simulink model "rbc_ut"  (Simulink 8.1)
settings: Solver=FixedStepDiscrete  StartTime=0.0  StopTime=Inf  FixedStep=0.005  RelTol=1e-3
PostLoadFcn:
  | , if any(exist('dsrtsu_mdlpostloadfcn', 'file') == [2, 3, 6]), try dsrtsu_mdlpostloadfcn('Execute', bdroot); catch fprintf('Error in PostLoadFcn (dsrtsu_mdlpostloadfcn) for model "%s":\n %s\n', bdroot, lasterr); end, end,
libraries: siltestlib x8, rbc x1
settings Model: DSRTSU_INTERNAL_RTI_VER=450  DSRTSU_INTERNAL_RTI_TYPE=rti1401  RTICANMMDATA=struct('GeneralSetupData',struct('modelroot','D:\ELN150201_TAIWAN\trunk\AdasDragon\software\sw_development\arch\app\acc','generalsettings',struct('filesettings',struct('destfolder',struct('Name','RTICANMM_FILES','Check',1),'buildfolder',struct('Name','.','Check',1),'AbsDestfolder',struct('Name','D:\ELN150201_TAIWAN\trunk\AdasDragon\software\sw_development\arch\app\acc\RTICANMM_FILES'),'AbsBuildfolder',struct('Name','D:\ELN150201_TAIWAN\trunk\AdasDragon\software\sw_development\arch\app\acc'))),'options',struct('addpaths',1,'rmpaths',1,'addtrcexclusion',logical(1),'cannavigator',struct('checkmonitoring',0),'show_usrtrc',0,'use_usrtrc',0),'advanced',struct('options',[1 1 1 1 1 1 1 1 1 1 1 1 1 1 1 1 1 1 1 1 1 1 1 1 1 1 1 1 1 1 1 1 1 1 1 1 1 1 1 1 1 1 1 1 1 1 1 1 1 1 1 1 1 1 1 1 1 1 1 1 1 1 1 1 1 1 1 1 1 1 1 1 1 1 1 1 1 1 1 1 1 1 1 1 1 1 1 1 1 1 1 1 1 1 1 1 1 1 1 1]),'MPSetup',{{}},'modelname','rbc_ut','block','rbc_ut'))  DSRTSU_INTERNAL_RTIFPGA=40  Creator=AT015411  LastModifiedBy=AT015555  BufferReuse=off
settings DataIOCC: SignalLoggingSaveFormat=Dataset
settings OptimizationCC: BlockReduction=off  OptimizeBlockIOStorage=off  BufferReuse=off  ExpressionFolding=off  ExpressionDepthLimit=128  LocalBlockOutputs=off
settings DebuggingCC: FcnCallInpInsideContextMsg=EnableAllAsError
settings HardwareCC: ProdIntDivRoundTo=Zero  ProdEndianess=BigEndian  ProdHWDeviceType=Generic->Custom  TargetIntDivRoundTo=Zero  TargetEndianess=BigEndian  TargetHWDeviceType=Generic->Custom
settings RTWCC: SystemTargetFile=rti1005.tlc  MakeCommand=make_rti  TemplateMakefile=rti1005.tmf  Description=dSPACE DS1005 Hardware Platform  ProcessScript=rti1005_make_rtw_hook
settings STFCustomTargetCC: CodeReplacementLibrary=ANSI_C  ParMdlRefBuildCompliant=on  GeneratePreprocessorConditionals=Disable all  MatFileLogging=on  SystemTargetFile=rti1005.tlc
settings GRTTargetCC: CompOptLevelCompliant=off  ConcurrentExecutionCompliant=off  ExtModeMexFile=noextcomm
settings CustomProperty: DataType=RTWOptions_EnumType_C__Program Files (x86)_dSPACE RCPHIL 2014-B_MATLAB_RTI_RTI1401_TLC_rti1005_1InitialSimState  Value=RUN
settings EnumStrPairs: String=RUN

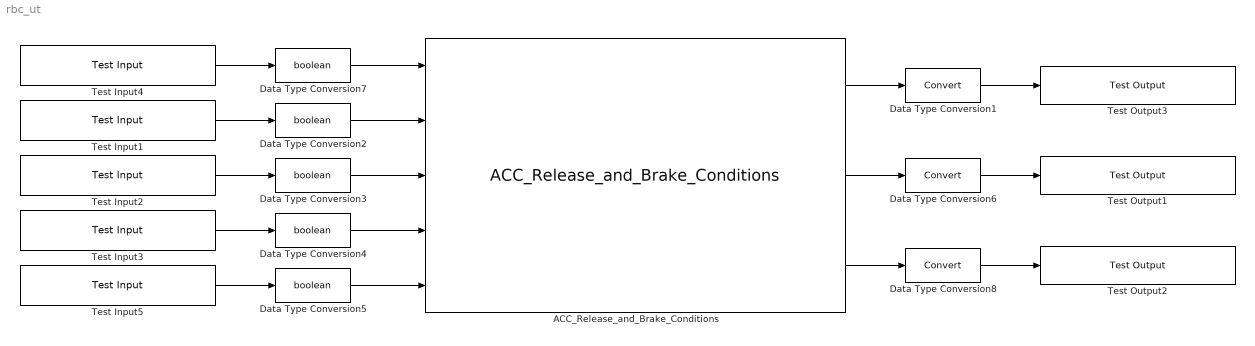
== system rbc_ut ==
  ACC_Release_and_Brake_Conditions : rbc/ACC_Release_and_Brake_Conditions
  Data Type Conversion1 : DataTypeConversion
  Data Type Conversion{2..5,7} (5 alike) : DataTypeConversion  OutDataTypeStr=boolean
  Data Type Conversion6 : DataTypeConversion
  Data Type Conversion8 : DataTypeConversion
  Test Input1 : siltestlib/Test Input  varname=VACC_ACCDecelControlEnable_flg  sampletime=0.005
  Test Input2 : siltestlib/Test Input  varname=VACC_ACCDecelControlDisable_flg  sampletime=0.005
  Test Input3 : siltestlib/Test Input  varname=VACC_ACCTransEnable_flg  sampletime=0.005
  Test Input4 : siltestlib/Test Input  varname=VACC_ACCSpdToBrake_flg  sampletime=0.005
  Test Input5 : siltestlib/Test Input  varname=VACC_ACCOverride_flg  sampletime=0.005
  Test Output1 : siltestlib/Test Output  varname=VACC_ACCStartBrake_flg  sampletime=-1
  Test Output2 : siltestlib/Test Output  varname=VACC_ACCEndBrake_flg  sampletime=-1
  Test Output3 : siltestlib/Test Output  varname=VACC_ACCStartRelease_flg  sampletime=-1
  wires:
  Data Type Conversion1/1 -> Test Output3/1
  ACC_Release_and_Brake_Conditions/1 -> Data Type Conversion1/1
  Test Input4/1 -> Data Type Conversion7/1
  Data Type Conversion7/1 -> ACC_Release_and_Brake_Conditions/1
  Test Input1/1 -> Data Type Conversion2/1
  Test Input2/1 -> Data Type Conversion3/1
  Test Input3/1 -> Data Type Conversion4/1
  Test Input5/1 -> Data Type Conversion5/1
  Data Type Conversion5/1 -> ACC_Release_and_Brake_Conditions/5
  Data Type Conversion2/1 -> ACC_Release_and_Brake_Conditions/2
  Data Type Conversion4/1 -> ACC_Release_and_Brake_Conditions/4
  Data Type Conversion3/1 -> ACC_Release_and_Brake_Conditions/3
  Data Type Conversion6/1 -> Test Output1/1
  Data Type Conversion8/1 -> Test Output2/1
  ACC_Release_and_Brake_Conditions/2 -> Data Type Conversion6/1
  ACC_Release_and_Brake_Conditions/3 -> Data Type Conversion8/1
